simulink model "MODELODETURBINADERIOV4"  (R2017a)
settings: Solver=ode1  StartTime=0.0  StopTime=4  FixedStep=50e-3  RelTol=1e-3
values from neighbouring files (symbols this model uses):
  A = pi()*((D/2)^2)    [MODELOHIDRO.m]    (also in MODELOHIDROV10.m; MODELOHIDROV2.m; MODELOHIDROV3.m; MODELOHIDROV4.m)
  B = 0    [MODELOHIDRO.m]    (also in MODELOHIDROV10.m; MODELOHIDROV2.m; MODELOHIDROV3.m; MODELOHIDROV4.m)
  beta = 0    [MODELOHIDRO.m]    (also in MODELOHIDROV10.m; MODELOHIDROV2.m; MODELOHIDROV3.m; MODELOHIDROV4.m)
  Bi = 0.2287    [MODELOHIDRO.m]    (also in MODELOHIDROV10.m = 0.1; MODELOHIDROV2.m; MODELOHIDROV3.m; MODELOHIDROV4.m = 0.005)
  den = 1000    [MODELOHIDRO.m]    (also in MODELOHIDROV10.m; MODELOHIDROV2.m; MODELOHIDROV3.m; MODELOHIDROV4.m)
  J = 16.1919e-4    (= 0.00161919)    [MODELOHIDROV10.m]    (also in MODELOHIDROV2.m = 100; MODELOHIDROV3.m = 10; MODELOHIDROV4.m; MODELOHIDROV7.m)
  Ji = 1    [MODELOHIDRO.m]    (also in MODELOHIDROV10.m = 1.72; MODELOHIDROV2.m; MODELOHIDROV3.m; MODELOHIDROV4.m = 0.0465)
  k = 1    [MODELOHIDRO.m]    (also in MODELOHIDROV2.m; MODELOHIDROV3.m)
  Kb = 1.8    [MODELOHIDRO.m]    (also in MODELOHIDROV10.m = 6.2; MODELOHIDROV2.m; MODELOHIDROV3.m; MODELOHIDROV4.m = 0.027)
  Kp = 0.4    [MODELOHIDRO.m]    (also in MODELOHIDROV10.m = 5.6627; MODELOHIDROV2.m; MODELOHIDROV3.m; MODELOHIDROV4.m = 0.027)
  m = 5    [MODELOHIDRO.m]    (also in MODELOHIDROV2.m; MODELOHIDROV3.m)
  r = D/2    (= 0.5)    [MODELOHIDRO.m]    (also in MODELOHIDROV10.m; MODELOHIDROV2.m; MODELOHIDROV3.m; MODELOHIDROV4.m)
  Ri = 0.6    [MODELOHIDRO.m]    (also in MODELOHIDROV10.m = 0.973; MODELOHIDROV2.m; MODELOHIDROV3.m; MODELOHIDROV4.m = 1)
  Rr = 5    [MODELOHIDROV4.m]    (also in MODELOHIDROV7.m; MODELOHIDROV8.m = 40)
  T_d = 0    [MODELOHIDRO.m]    (also in MODELOHIDROV10.m; MODELOHIDROV2.m; MODELOHIDROV3.m; MODELOHIDROV4.m)
  z = 2    [MODELOHIDRO.m]    (also in MODELOHIDROV2.m; MODELOHIDROV3.m)
undefined symbols (not defined in the file or in its folder): CDC, DDC, LDC, RDC, sigbuilder_block
libraries: powerlib x17, powerlib_meascontrol x2, simulink x1
settings Model: Creator=zni.uao  LastModifiedBy=zni.uao

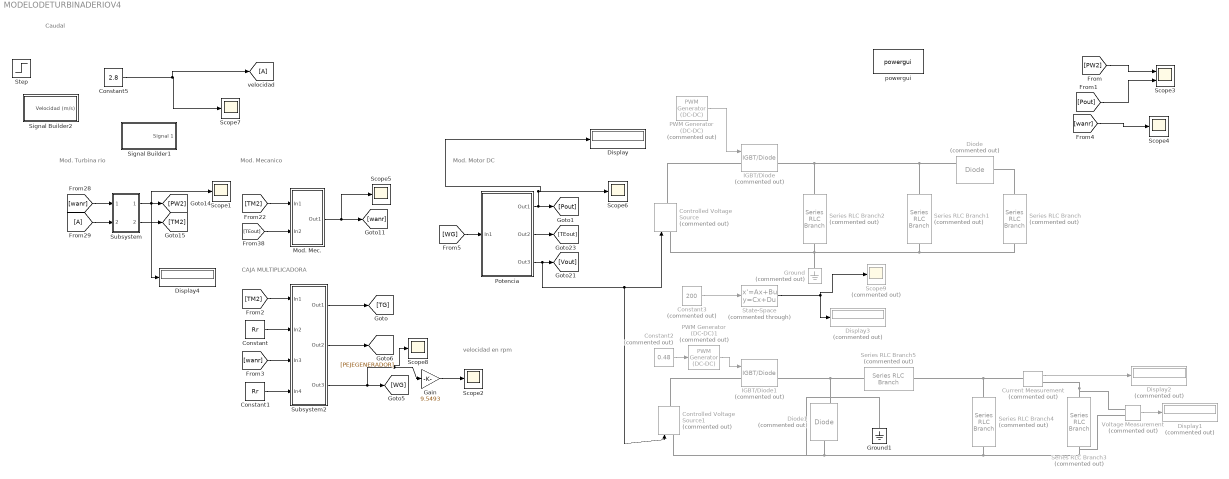
== system MODELODETURBINADERIOV4 ==
  note: velocidad en rpm
  note: CAJA MULTIPLICADORA
  note: Mod. Motor DC
  note: Mod. Turbina rio
  note: Mod. Mecanico
  note: Caudal
  Constant : Constant  Value=Rr
  Constant1 : Constant  Value=Rr
  Constant2 : Constant  Commented=on  Value=0.48
  Constant3 : Constant  Commented=on  Value=200
  Constant5 : Constant  Value=2.8
  Controlled Voltage Source : powerlib/Electrical Sources/Controlled Voltage Source  Commented=on  Initialize=on  Source_Type=AC  Amplitude=0  Phase=0  Frequency=0  Measurements=None
  Controlled Voltage Source1 : powerlib/Electrical Sources/Controlled Voltage Source  Commented=on  Initialize=on  Source_Type=DC  Amplitude=0  Phase=0  Frequency=0  Measurements=None
  Current Measurement : powerlib/Measurements/Current Measurement  Commented=on  PhasorSimulation=off  OutputType=Complex  PSBequivalent=0
  Diode : powerlib/Power Electronics/Diode  Commented=on  Ron=0.001  Lon=0  Vf=0.8  IC=0  UseSnubber=0  Rs=500  Cs=250e-9  Measurements=on
  Diode1 : powerlib/Power Electronics/Diode  Commented=on  Ron=0.001  Lon=0  Vf=0.8  IC=0  UseSnubber=0  Rs=500  Cs=250e-9  Measurements=on
  Display : Display
  Display1 : Display  Commented=on
  Display2 : Display  Commented=on
  Display3 : Display  Commented=on
  Display4 : Display
  Gain : Gain  Gain=9.5493
  Ground : powerlib/Elements/Ground  Commented=on  LConnTagsString=a
  Ground1 : powerlib/Elements/Ground  LConnTagsString=a
  IGBT/Diode : powerlib/Power Electronics/IGBT//Diode  Commented=on  Ron=1e-3  Rs=1e5  Cs=inf  Measurements=on
  IGBT/Diode1 : powerlib/Power Electronics/IGBT//Diode  Commented=on  Ron=1e-3  Rs=1e5  Cs=inf  Measurements=on
  Mod. Mec. : Subsystem
  PWM Generator (DC-DC) : powerlib_meascontrol/Pulse & Signal Generators/PWM Generator (DC-DC)  Commented=on  Fsw=5000  Ts=0
  PWM Generator (DC-DC)1 : powerlib_meascontrol/Pulse & Signal Generators/PWM Generator (DC-DC)  Commented=on  Fsw=20000  Ts=0.05
  Potencia : Subsystem
  Scope{1..2,4..8} (7 alike) : Scope
  Scope3 : Scope  NumInputPorts=2
  Scope9 : Scope  Commented=on
  Series RLC Branch : powerlib/Elements/Series RLC Branch  Commented=on  LConnTagsString=__new0  RConnTagsString=__new0  BranchType=R  Resistance=1  Inductance=1e-3  SetiL0=off  InitialCurrent=0  Capacitance=1e-6  Setx0=off  InitialVoltage=0  Measurements=None
  Series RLC Branch1 : powerlib/Elements/Series RLC Branch  Commented=on  LConnTagsString=__new0  RConnTagsString=__new0  BranchType=C  Resistance=1  Inductance=1e-3  SetiL0=off  InitialCurrent=0  Capacitance=1e-6  Setx0=off  InitialVoltage=0  Measurements=None
  Series RLC Branch2 : powerlib/Elements/Series RLC Branch  Commented=on  LConnTagsString=__new0  RConnTagsString=__new0  BranchType=L  Resistance=1  Inductance=1e-3  SetiL0=off  InitialCurrent=0  Capacitance=1e-6  Setx0=off  InitialVoltage=0  Measurements=None
  Series RLC Branch3 : powerlib/Elements/Series RLC Branch  Commented=on  LConnTagsString=__new0  RConnTagsString=__new0  BranchType=R  Resistance=6.44  Inductance=1e-3  SetiL0=off  InitialCurrent=0  Capacitance=1e-6  Setx0=off  InitialVoltage=0  Measurements=None
  Series RLC Branch4 : powerlib/Elements/Series RLC Branch  Commented=on  LConnTagsString=__new0  RConnTagsString=__new0  BranchType=C  Resistance=1  Inductance=1e-3  SetiL0=off  InitialCurrent=0  Capacitance=2.91e-3  Setx0=off  InitialVoltage=0  Measurements=None
  Series RLC Branch5 : powerlib/Elements/Series RLC Branch  Commented=on  LConnTagsString=__new0  RConnTagsString=__new0  BranchType=L  Resistance=1  Inductance=83.72e-6  SetiL0=off  InitialCurrent=0  Capacitance=1e-6  Setx0=off  InitialVoltage=0  Measurements=None
  Signal Builder1 : Subsystem  Tag=STV Subsys  LoadFcn=sigbuilder_block('load');  StartFcn=sigbuilder_block('start');  StopFcn=sigbuilder_block('stop');  ClipboardFcn=sigbuilder_block('clipboard');  mask(Sigbuilder block){tuvar=[0:10]}
      mask help: Simulink:masks:SigbuilderBlock_MD
      mask init:
      | if ~strcmp(get_param(bdroot(gcbh),'SimulationStatus'),'stopped') tuvar = sigbuilder_block('maskInit'); end
      settings: CopyFcn=sigbuilder_block('copy');  DeleteFcn=sigbuilder_block('delete');  ModelCloseFcn=sigbuilder_block('modelClose');  PreSaveFcn=sigbuilder_block('preSave');  PauseFcn=sigbuilder_block('pause');  ContinueFcn=sigbuilder_block('continue');  NameChangeFcn=sigbuilder_block('namechange');  OpenFcn=sigbuilder_block('open',[211.5 75 550.5 359.25 ]);  CloseFcn=sigbuilder_block('close');
      mask Display: plot(0, 0, 100, 100,[2, 2, 32, 32, 2], [68, 8, 8, 68, 68],[32, 2], [38, 38], [32, 19, 2],[53, 60, 44], [32, 17, 17, 2],[16, 16, 31, 31]);txt = getActiveGroup(gcbh);text(2, 100, txt,'verticalAlignment', 'top');
  Signal Builder2 : Subsystem  Tag=STV Subsys  LoadFcn=sigbuilder_block('load');  StartFcn=sigbuilder_block('start');  StopFcn=sigbuilder_block('stop');  ClipboardFcn=sigbuilder_block('clipboard');  mask(Sigbuilder block){tuvar=[0:10]}
      mask help: Simulink:masks:SigbuilderBlock_MD
      mask init:
      | if ~strcmp(get_param(bdroot(gcbh),'SimulationStatus'),'stopped') tuvar = sigbuilder_block('maskInit'); end
      settings: CopyFcn=sigbuilder_block('copy');  DeleteFcn=sigbuilder_block('delete');  ModelCloseFcn=sigbuilder_block('modelClose');  PreSaveFcn=sigbuilder_block('preSave');  PauseFcn=sigbuilder_block('pause');  ContinueFcn=sigbuilder_block('continue');  NameChangeFcn=sigbuilder_block('namechange');  OpenFcn=sigbuilder_block('open',[197.25 66 550.5 359.25 ]);  CloseFcn=sigbuilder_block('close');
      mask Display: plot(0, 0, 100, 100,[2, 2, 32, 32, 2], [68, 8, 8, 68, 68],[32, 2], [38, 38], [32, 19, 2],[53, 60, 44], [32, 17, 17, 2],[16, 16, 31, 31]);txt = getActiveGroup(gcbh);text(2, 100, txt,'verticalAlignment', 'top');
  State-Space : StateSpace  Commented=through  A=[0 (-1/LDC);(1/CDC) -(1/(RDC*CDC))]  B=[(DDC/LDC);0]  C=[0 1]  D=0  X0=0
  Step : Step  Time=10  Before=2.5  After=2.888  SampleTime=0
  Subsystem : Subsystem
  Subsystem2 : Subsystem
  Voltage Measurement : powerlib/Measurements/Voltage Measurement  Commented=on  PhasorSimulation=off  OutputType=Complex  PSBequivalent=0
  powergui : powerlib/powergui  Priority=1  SimulationMode=Discrete  SampleTime=50e-3  frequency=60  Iterations=50  frequencyindice=60  Pbase=100e6  ErrMax=1e-4  UnitsV=kV  UnitsW=MW  buscounter=0  FunctionMessages=off  echomessages=off  EnableUseOfTLC=off  CurrentSourceSwitches=off  DisableSnubberDevices=off  DisableRonSwitches=off  DisableVfSwitches=off  DisplayEquations=off  SolverType=Tustin/Backward Euler (TBE)  Interpol=off  ExternalGateDelay=off  methode=off  Ts=100  x0status=blocks  SPID=off  SwTol=0  HookPort=off  RestoreLinks=warning  ResistiveCurrentMeasurement=off  Frange=[0:2:500]  Ylog=off  Xlog=on  ShowGrid=off  save=off  variable=ZData  structure=0  ZoomFFT=off  StartTime=0.0  cycles=1  DisplayStyle=1  fundamental=60  FreqAxis=off  MaxFrequency=1000  frequencyindicesteady=0 Hz  RmsSteady=1  display=off
  wires:
  [wanr] -> Subsystem/1(In1)
  [A] -> Subsystem/2(In2)
  Subsystem/1(Out1) -> Display4/1, Scope1/1, [PW2]
  Subsystem/2(Out2) -> [TM2]
  Mod. Mec./1(Out1) -> Scope5/1, [wanr]
  [TM2] -> Mod. Mec./1(In1)
  Potencia/1(Out1) -> Display/1, Scope6/1, [Pout]
  Potencia/2(Out2) -> [TEout]
  [TEout] -> Mod. Mec./2(In2)
  [TM2] -> Subsystem2/1(In1)
  Constant/1 -> Subsystem2/2(In2)
  [wanr] -> Subsystem2/3(In3)
  Constant1/1 -> Subsystem2/4(In4)
  Subsystem2/1(Out1) -> [TG]
  Subsystem2/2(Out2) -> [PEJEGENERADOR]
  Subsystem2/3(Out3) -> Scope8/1, Gain/1, [WG]
  Gain/1 -> Scope2/1
  [WG] -> Potencia/1(In1)
  [PW2] -> Scope3/1
  [Pout] -> Scope3/2
  [wanr] -> Scope4/1
  Constant5/1 -> [A], Scope7/1
  Potencia/3(Out3) -> Controlled Voltage Source1/1, Controlled Voltage Source/1, [Vout]
  PWM Generator (DC-DC)/1 -> IGBT/Diode/1
  PWM Generator (DC-DC)1/1 -> IGBT/Diode1/1
  Constant2/1 -> PWM Generator (DC-DC)1/1
  Voltage Measurement/1 -> Display1/1
  Current Measurement/1 -> Display2/1
  State-Space/1 -> Scope9/1, Display3/1
  Constant3/1 -> State-Space/1
  connections:
  Series RLC Branch/LConn1 -- Diode/LConn1
  Diode/RConn1 -- IGBT/Diode/RConn1 -- Series RLC Branch2/LConn1 -- Series RLC Branch1/LConn1
  Series RLC Branch2/RConn1 -- Ground/LConn1 -- Controlled Voltage Source/LConn1 -- Series RLC Branch/RConn1 -- Series RLC Branch1/RConn1
  Controlled Voltage Source/RConn1 -- IGBT/Diode/LConn1
  Diode1/LConn1 -- Controlled Voltage Source1/LConn1 -- Series RLC Branch4/RConn1 -- Voltage Measurement/LConn2 -- Series RLC Branch3/RConn1 -- Ground1/LConn1
  Series RLC Branch5/LConn1 -- Current Measurement/LConn1 -- Series RLC Branch4/LConn1
  Series RLC Branch5/RConn1 -- IGBT/Diode1/RConn1 -- Diode1/RConn1
  IGBT/Diode1/LConn1 -- Controlled Voltage Source1/RConn1
  Current Measurement/RConn1 -- Voltage Measurement/LConn1 -- Series RLC Branch3/LConn1

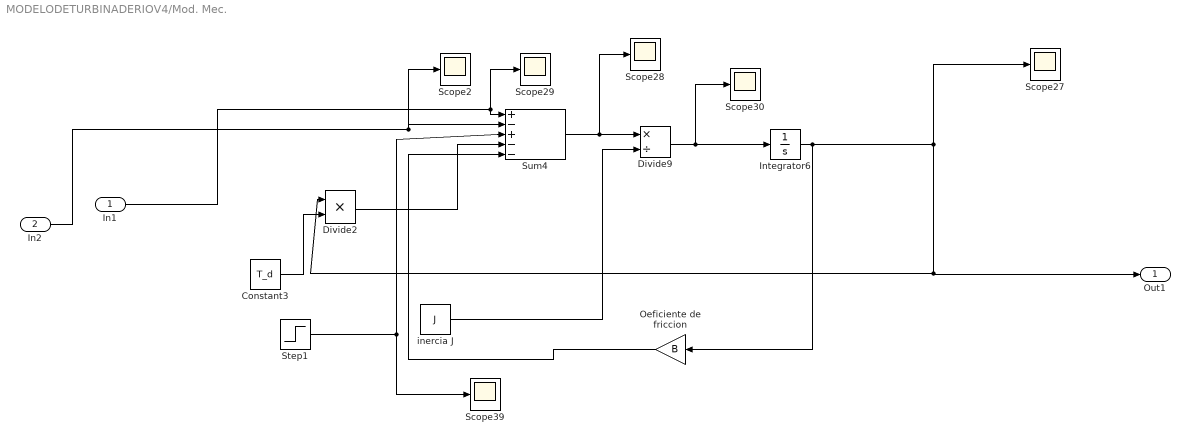
== system MODELODETURBINADERIOV4/Mod. Mec. ==
  In1 : Inport
  In2 : Inport  Port=2
  Constant3 : Constant  Value=T_d
  Divide2 : Product  Inputs=**
  Divide9 : Product  Inputs=*/
  Integrator6 : Integrator  InitialCondition=10
  Oeficiente de friccion : Gain  Gain=B
  Scope{2,27..30,39} (6 alike) : Scope
  Step1 : Step  Time=3  Before=5  After=0  SampleTime=0
  Sum4 : Sum  Inputs=|+-+--
  inercia J : Constant  Value=J
  Out1 : Outport
  wires:
  inercia J/1 -> Divide9/2
  Constant3/1 -> Divide2/2
  Divide2/1 -> Sum4/4
  Oeficiente de friccion/1 -> Sum4/5
  Step1/1 -> Scope39/1, Sum4/3
  Sum4/1 -> Scope28/1, Divide9/1
  In1/1 -> Scope29/1, Sum4/1
  In2/1 -> Scope2/1, Sum4/2
  Divide9/1 -> Scope30/1, Integrator6/1
  Integrator6/1 -> Out1/1, Divide2/1, Scope27/1, Oeficiente de friccion/1

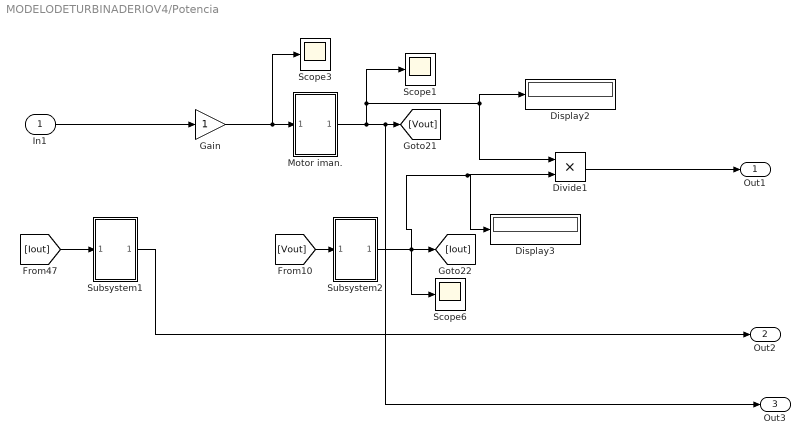
== system MODELODETURBINADERIOV4/Potencia ==
  In1 : Inport
  Display2 : Display
  Display3 : Display
  Divide1 : Product  Inputs=**
  Gain : Gain
  Motor iman. : Subsystem
  Scope1 : Scope
  Scope3 : Scope
  Scope6 : Scope
  Subsystem1 : Subsystem
  Subsystem2 : Subsystem
  Out1 : Outport
  Out2 : Outport  Port=2
  Out3 : Outport  Port=3
  wires:
  Motor iman./1(Out1) -> Out3/1, [Vout], Scope1/1, Divide1/1, Display2/1
  Subsystem1/1(Out1) -> Out2/1
  [Iout] -> Subsystem1/1(In1)
  Subsystem2/1(Out1) -> Divide1/2, Display3/1, Scope6/1, [Iout]
  Divide1/1 -> Out1/1
  Gain/1 -> Scope3/1, Motor iman./1(In1)
  In1/1 -> Gain/1
  [Vout] -> Subsystem2/1(In1)

== system MODELODETURBINADERIOV4/Signal Builder1 ==
  Demux : Demux  Tag=STV Demux  Outputs=1
  FromWs : FromWorkspace  Tag=STV FromWs  VariableName=tuvar  SampleTime=0
      SigBuilderData=|
      | common.afterFinalStr = 'Extrapolate'
      | common.sampleTime = 0
      | dataSet.timeRange = [0 200]
      | dataSet.name = 'Group 1'
      | sbobj.Groups.Name = 'Group 1'
      | sbobj.Groups.Signals.Name = 'Signal 1'
      | sbobj.Groups.Signals.XData = [0 1.25 2.5 3.75 5 6.25 7.5 8.75 10 11.25 12.5 13.75 15 16.25 17.5 18.75 20 21.25 22.5 23.75 25 26.25 27.5 28.75 30 31.25 32.5 33.75 35 36.25 37.5 38.75 40 41.25 42.5 43.75 45 46.25 47.5 48.75 50 51.25 52.5 53.75 55 56.25 57.5 58.75 60 61.25 62.5 63.75 65 66.25 67.5 68.75 70 71.25 72.5 73.75 75 76.25 77.5 78.75 80 81.25 82.5 83.75 85 86.25 87.5 88.75 90 91.25 92.5 93.75 93.75 95 95 96.25 97.5 98.75 100 101.25 102.5 103.75 105 106.25 107.5 108.75 110 111.25 112.5 113.75 115 116.25 117.5 118.75 120 121.25 122.5 123.75 125 126.25 127.5 128.75 130 131.25 132.5 133.75 135 136.25 137.5 138.75 140 141.25 142.5 143.75 145 146.25 147.5 148.75 150 151.25 152.5 153.75 155 156.25 157.5 158.75 160 161.25 162.5 163.75 165 166.25 167.5 168.75 170 171.25 172.5 173.75 175 176.25 177.5 178.75 180 181.25 182.5 183.75 185 186.25 187.5 188.75 190 191.25 192.5 193.75 195 196.25 197.5 198.75 200]
      | sbobj.Groups.Signals.YData = [2.6 2.67071067812 2.7 2.67071067812 2.6 2.52928932188 2.5 2.52928932188 2.6 2.67071067812 2.7 2.67071067812 2.6 2.52928932188 2.5 2.52928932188 2.6 2.67071067812 2.7 2.67071067812 2.6 2.52928932188 2.5 2.52928932188 2.6 2.67071067812 2.7 2.67071067812 2.6 2.52928932188 2.5 2.52928932188 2.6 2.67071067812 2.7 2.67071067812 2.6 2.52928932188 2.5 2.52928932188 2.6 2.67071067812 2.7 2.67071067812 2.6 2.52928932188 2.5 2.52928932188 2.6 2.67071067812 2.7 2.67071067812 2.6 2.52928932188 2.5 2.52928932188 2.6 2.67071067812 2.7 2.67071067812 2.6 2.52928932188 2.5 2.52928932188 2.6 2.67071067812 2.7 2.67071067812 2.6 2.52928932188 2.5 2.52928932188 2.6 2.67071067812 2.7 2.67071067812 2.67071067812 2.6 2.6 2.52928932188 2.5 2.52928932188 2.6 2.67071067812 2.7 2.67071067812 2.6 2.52928932188 2.5 2.52928932188 2.6 2.67071067812 2.7 2.67071067812 2.6 2.52928932188 2.5 2.52928932188 2.6 2.67071067812 2.7 2.67071067812 2.6 2.52928932188 2.5 2.52928932188 2.6 2.67071067812 2.7 2.67071067812 2.6 2.52928932188 2.5 2.52928932188 2.6 2.67071067812 2.7 2.67071067812 2.6 2.52928932188 2.5 2.52928932188 2.6 2.67071067812 2.7 2.67071067812 2.6 2.52928932188 2.5 2.52928932188 2.6 2.67071067812 2.7 2.67071067812 2.6 2.52928932188 2.5 2.52928932188 2.6 2.67071067812 2.7 2.67071067812 2.6 2.52928932188 2.5 2.52928932188 2.6 2.67071067812 2.7 2.67071067812 2.6 2.52928932188 2.5 2.52928932188 2.6 2.67071067812 2.7 2.67071067812 2.6 2.52928932188 2.5 2.52928932188 2.6]
      | sbobj.Groups.TimeRange = [0 200]
  Signal 1 : Outport  Tag=STV Outport
  wires:
  FromWs/1 -> Demux/1
  Demux/1 -> Signal 1/1

== system MODELODETURBINADERIOV4/Signal Builder2 ==
  Demux : Demux  Tag=STV Demux  Outputs=1
  FromWs : FromWorkspace  Tag=STV FromWs  VariableName=tuvar  SampleTime=0
      SigBuilderData=|
      | common.afterFinalStr = 'Extrapolate'
      | common.sampleTime = 0
      | dataSet.timeRange = [0 200]
      | dataSet.name = 'Group 1'
      | sbobj.Groups.Name = 'Group 1'
      | sbobj.Groups.Signals.Name = 'Velocidad (m/s)'
      | sbobj.Groups.Signals.XData = [0 120 120 180.5 180.5 200]
      | sbobj.Groups.Signals.YData = [2 2 2.5 2.5 2.8 2.8]
      | sbobj.Groups.TimeRange = [0 200]
  Velocidad (m/s) : Outport  Tag=STV Outport
  wires:
  FromWs/1 -> Demux/1
  Demux/1 -> Velocidad (m/s)/1

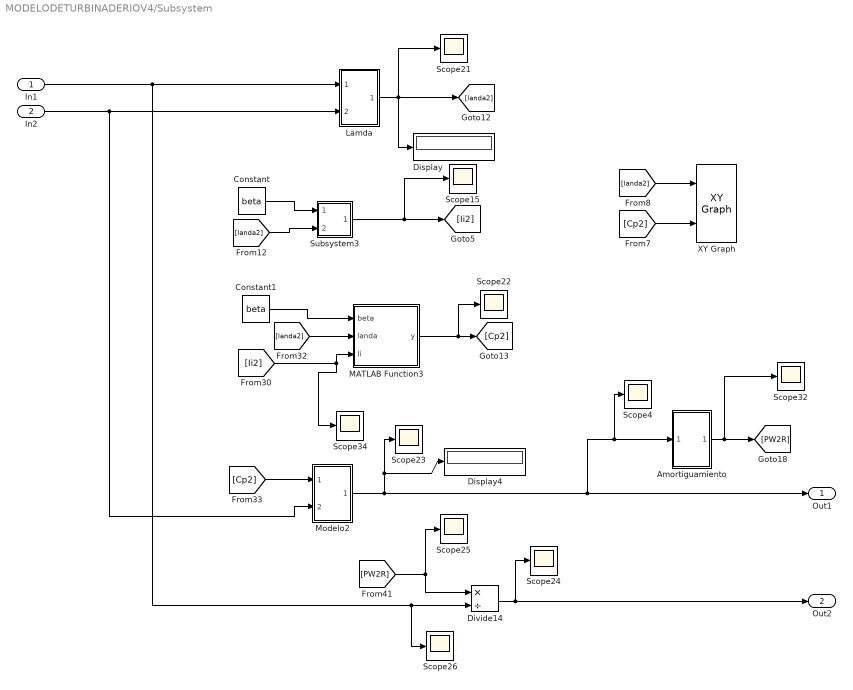
== system MODELODETURBINADERIOV4/Subsystem ==
  In1 : Inport
  In2 : Inport  Port=2
  Amortiguamiento : Subsystem
  Constant : Constant  Value=beta
  Constant1 : Constant  Value=beta
  Display : Display
  Display4 : Display
  Divide14 : Product  Inputs=*/
  Lamda : Subsystem
  MATLAB Function3 : MATLAB Function  TreatAsAtomicUnit=on
  Modelo2 : Subsystem
  Scope{4,15,21..26,32,34} (10 alike) : Scope
  Subsystem3 : Subsystem
  XY Graph : simulink/Sinks/XY Graph  xmin=1  xmax=20  ymin=0  ymax=0.56  st=0.1
  Out1 : Outport
  Out2 : Outport  Port=2
  wires:
  Modelo2/1(Out1) -> Amortiguamiento/1(In1), Scope4/1, Out1/1, Display4/1, Scope23/1
  Constant1/1 -> MATLAB Function3/1(beta)
  Divide14/1 -> Out2/1, Scope24/1
  [Ii2] -> Scope34/1, MATLAB Function3/3(Ii)
  [Cp2] -> Modelo2/1(In1)
  [PW2R] -> Scope25/1, Divide14/1
  In1/1 -> Scope26/1, Divide14/2, Lamda/1(In1)
  [landa2] -> MATLAB Function3/2(landa)
  In2/1 -> Modelo2/2(In2), Lamda/2(In2)
  Lamda/1(Out1) -> Display/1, [landa2], Scope21/1
  MATLAB Function3/1(y) -> Scope22/1, [Cp2]
  [landa2] -> XY Graph/1
  Constant/1 -> Subsystem3/1(In1)
  [landa2] -> Subsystem3/2(In2)
  Amortiguamiento/1(Out1) -> Scope32/1, [PW2R]
  Subsystem3/1(Out1) -> Scope15/1, [Ii2]
  [Cp2] -> XY Graph/2

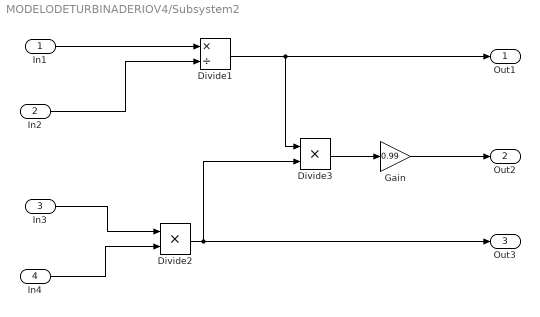
== system MODELODETURBINADERIOV4/Subsystem2 ==
  In1 : Inport
  In2 : Inport  Port=2
  In3 : Inport  Port=3
  In4 : Inport  Port=4
  Divide1 : Product  Inputs=*/
  Divide2 : Product  Inputs=**
  Divide3 : Product  Inputs=**
  Gain : Gain  Gain=0.99
  Out1 : Outport
  Out2 : Outport  Port=2
  Out3 : Outport  Port=3
  wires:
  Gain/1 -> Out2/1
  In1/1 -> Divide1/1
  Divide2/1 -> Out3/1, Divide3/2
  In3/1 -> Divide2/1
  In4/1 -> Divide2/2
  Divide1/1 -> Out1/1, Divide3/1
  In2/1 -> Divide1/2
  Divide3/1 -> Gain/1

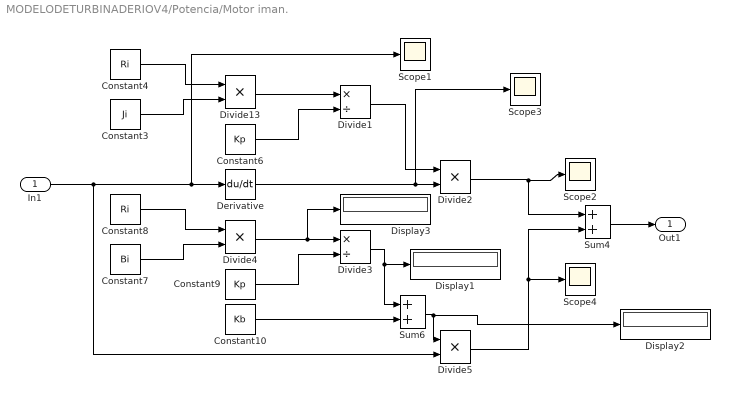
== system MODELODETURBINADERIOV4/Potencia/Motor iman. ==
  In1 : Inport
  Constant10 : Constant  Value=Kb
  Constant3 : Constant  Value=Ji
  Constant4 : Constant  Value=Ri
  Constant6 : Constant  Value=Kp
  Constant7 : Constant  Value=Bi
  Constant8 : Constant  Value=Ri
  Constant9 : Constant  Value=Kp
  Derivative : Derivative
  Display1 : Display
  Display2 : Display
  Display3 : Display
  Divide1 : Product  Inputs=*/  SaturateOnIntegerOverflow=on  RndMeth=Zero
  Divide{2,4..5,13} (4 alike) : Product  Inputs=**  SaturateOnIntegerOverflow=on  RndMeth=Zero
  Divide3 : Product  Inputs=*/  SaturateOnIntegerOverflow=on  RndMeth=Zero
  Scope{1..4} (4 alike) : Scope
  Sum4 : Sum
  Sum6 : Sum
  Out1 : Outport
  wires:
  Constant10/1 -> Sum6/2
  Divide2/1 -> Scope2/1, Sum4/1
  In1/1 -> Divide5/2, Scope1/1, Derivative/1
  Divide3/1 -> Display1/1, Sum6/1
  Divide13/1 -> Divide1/1
  Constant6/1 -> Divide1/2
  Constant4/1 -> Divide13/1
  Sum6/1 -> Display2/1, Divide5/1
  Divide1/1 -> Divide2/1
  Constant3/1 -> Divide13/2
  Constant9/1 -> Divide3/2
  Divide4/1 -> Display3/1, Divide3/1
  Constant7/1 -> Divide4/2
  Constant8/1 -> Divide4/1
  Derivative/1 -> Scope3/1, Divide2/2
  Sum4/1 -> Out1/1
  Divide5/1 -> Scope4/1, Sum4/2

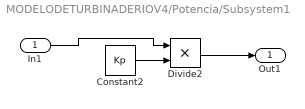
== system MODELODETURBINADERIOV4/Potencia/Subsystem1 ==
  In1 : Inport
  Constant2 : Constant  Value=Kp
  Divide2 : Product  Inputs=**
  Out1 : Outport
  wires:
  In1/1 -> Divide2/1
  Constant2/1 -> Divide2/2
  Divide2/1 -> Out1/1

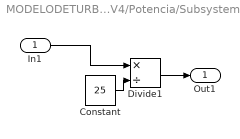
== system MODELODETURBINADERIOV4/Potencia/Subsystem2 ==
  In1 : Inport
  Constant : Constant  Value=25
  Divide1 : Product  Inputs=*/
  Out1 : Outport
  wires:
  Divide1/1 -> Out1/1
  Constant/1 -> Divide1/2
  In1/1 -> Divide1/1

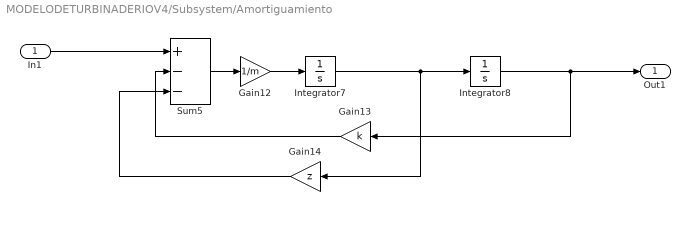
== system MODELODETURBINADERIOV4/Subsystem/Amortiguamiento ==
  In1 : Inport
  Gain12 : Gain  Gain=1/m
  Gain13 : Gain  Gain=k
  Gain14 : Gain  Gain=z
  Integrator7 : Integrator
  Integrator8 : Integrator
  Sum5 : Sum  Inputs=+--
  Out1 : Outport
  wires:
  Gain13/1 -> Sum5/2
  Integrator8/1 -> Out1/1, Gain13/1
  Integrator7/1 -> Gain14/1, Integrator8/1
  Sum5/1 -> Gain12/1
  Gain12/1 -> Integrator7/1
  Gain14/1 -> Sum5/3
  In1/1 -> Sum5/1

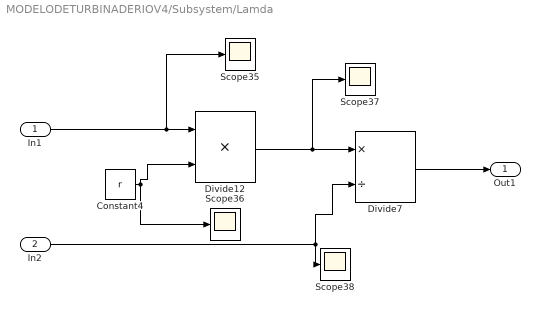
== system MODELODETURBINADERIOV4/Subsystem/Lamda ==
  In1 : Inport
  In2 : Inport  Port=2
  Constant4 : Constant  Value=r
  Divide12 : Product  Inputs=**
  Divide7 : Product  Inputs=*/
  Scope{35..38} (4 alike) : Scope
  Out1 : Outport
  wires:
  Divide7/1 -> Out1/1
  Constant4/1 -> Divide12/2, Scope36/1
  In2/1 -> Divide7/2, Scope38/1
  Divide12/1 -> Scope37/1, Divide7/1
  In1/1 -> Scope35/1, Divide12/1

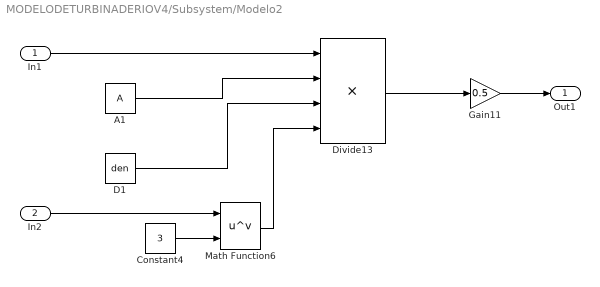
== system MODELODETURBINADERIOV4/Subsystem/Modelo2 ==
  In1 : Inport
  In2 : Inport  Port=2
  A1 : Constant  Value=A
  Constant4 : Constant  Value=3
  D1 : Constant  Value=den
  Divide13 : Product  Inputs=****  SaturateOnIntegerOverflow=on  RndMeth=Zero
  Gain11 : Gain  Gain=0.5
  Math Function6 : Math  Operator=pow  SaturateOnIntegerOverflow=on
  Out1 : Outport
  wires:
  Constant4/1 -> Math Function6/2
  Divide13/1 -> Gain11/1
  D1/1 -> Divide13/3
  In1/1 -> Divide13/1
  Gain11/1 -> Out1/1
  A1/1 -> Divide13/2
  In2/1 -> Math Function6/1
  Math Function6/1 -> Divide13/4

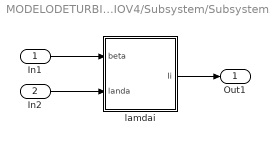
== system MODELODETURBINADERIOV4/Subsystem/Subsystem3 ==
  In1 : Inport
  In2 : Inport  Port=2
  lamdai : MATLAB Function  TreatAsAtomicUnit=on
  Out1 : Outport
  wires:
  lamdai/1(Ii) -> Out1/1
  In2/1 -> lamdai/2(landa)
  In1/1 -> lamdai/1(beta)

== matlab function MODELODETURBINADERIOV4/Subsystem/MATLAB Function3 ==
  data: beta input; y output; landa input; Ii input
function y = fcn(beta, landa,Ii)
w=0.5176; 
w1=116/Ii;
 w2=0.4*beta;
 w3=exp(-21/Ii);
 
 cp=w*(w1-w2-5)*w3+0.0068*landa;
 
 
 
 
 
y=cp;

== matlab function MODELODETURBINADERIOV4/Subsystem/Subsystem3/lamdai ==
  data: beta input; Ii output; landa input
function Ii = fcn(beta,landa)


Iii=(1/((landa+(0.08*beta))))-((0.035)/((beta^3)+1));
Ii=1/Iii;
